simulink model "simL0_multiPath"  (R2024a)
settings: Solver=ode4  StartTime=0.0  StopTime=1500  FixedStep=0.01  MaxStep=0.01  MinStep=10^-3  RelTol=0.01
values from neighbouring files (symbols this model uses):
  MegAWESkite = yaml.ReadYaml('MegAWESkite.yaml',false,true)    [runMain.m]
undefined symbols (not defined in the file or in its folder): actuatorLimit, controllerGains_retraction, controllerGains_traction, DiscIntNeverNeededParam, ENVMT, pathparam, simInit, tetherParams, winchParameter
libraries: simulink x9, slpidlib x9, sharedtransform x3, aerolibutil x3, dspswit3 x2, dspinverses x2, shared6dof x1, simulink_extras x1, dspsigops x1, dspstat3 x1, vrlib x1
(part 3 of 5)

== system simL0_multiPath/Controls/RatesControl/rate controller/Pitch ==
  In1 : Inport
  In2 : Inport  Port=2
  Divide2 : Product  Inputs=*/
  Multiport Switch : MultiPortSwitch  SaturateOnIntegerOverflow=off  InputSameDT=off
  PID Controller : slpidlib/PID Controller  Controller=P  Form=Parallel  TimeDomain=Continuous-time  UseExternalTs=off  SampleTime=-1  IntegratorMethod=Forward Euler  FilterMethod=Forward Euler  ControllerParametersSource=internal  P=controllerGains_traction.ratePitch_P  I=1  UseKiTs=off  D=0  UseExternalDerivativeSource=off  N=100  UseFilter=on  TunerSelectOption=Transfer Function Based (PID Tuner App)  InitialConditionSource=internal  InitialConditionForIntegrator=0  InitialConditionForFilter=0  DifferentiatorICPrevScaledInput=0  ExternalReset=none  TrackingMode=off  Kt=1  LimitOutput=off  SatLimitsSource=internal  UpperSaturationLimit=inf  LowerSaturationLimit=-inf  LinearizeAsGain=on  AntiWindupMode=none  Kb=1  LimitIntegrator=off  UpperIntegratorSaturationLimit=inf  LowerIntegratorSaturationLimit=-inf  POutMin=[]  POutMax=[]  IOutMin=[]  IOutMax=[]  DOutMin=[]  DOutMax=[]  NOutMin=[]  NOutMax=[]  SumOutMin=[]  SumOutMax=[]  SaturationOutMin=[]  SaturationOutMax=[]  PParamMin=[]  PParamMax=[]  IParamMin=[]  IParamMax=[]  DParamMin=[]  DParamMax=[]  NParamMin=[]  NParamMax=[]  KbParamMin=[]  KbParamMax=[]  KtParamMin=[]  KtParamMax=[]  KbOutMin=[]  KbOutMax=[]  KtOutMin=[]  KtOutMax=[]  IntegratorOutMin=[]  IntegratorOutMax=[]  FilterOutMin=[]  FilterOutMax=[]  SumI1OutMin=[]  SumI1OutMax=[]  SumI2OutMin=[]  SumI2OutMax=[]  SumI3OutMin=[]  SumI3OutMax=[]  SumI4OutMin=[]  SumI4OutMax=[]  SumDOutMin=[]  SumDOutMax=[]  DifferentiatorOutMin=[]  DifferentiatorOutMax=[]  FilterDiffOutCoefMin=[]  FilterDiffOutCoefMax=[]  ReciprocalOutMin=[]  ReciprocalOutMax=[]  SumDenOutMin=[]  SumDenOutMax=[]  SumNumOutMin=[]  SumNumOutMax=[]  DivideOutMin=[]  DivideOutMax=[]  UdiffTsProdOutMin=[]  UdiffTsProdOutMax=[]  NTsProdOutMin=[]  NTsProdOutMax=[]  UintegralTsProdOutMin=[]  UintegralTsProdOutMax=[]  UngainTsProdOutMin=[]  UngainTsProdOutMax=[]  ClampingZeroOutDataTypeStr=Inherit: Inherit via back propagation  ClampingZeroOutMin=[]  ClampingZeroOutMax=[]  FilterDenConstantOutDataTypeStr=Inherit: Inherit via back propagation  FilterDenConstantOutMin=[]  FilterDenConstantOutMax=[]  PCopyOutDataTypeStr=Inherit: Inherit via back propagation  PCopyOutMin=[]  PCopyOutMax=[]  NCopyOutDataTypeStr=Inherit: Inherit via back propagation  NCopyOutMin=[]  NCopyOutMax=[]  IntegratorContinuousStateAttributes=''  IntegratorStateMustResolveToSignalObject=off  IntegratorRTWStateStorageClass=Auto  FilterContinuousStateAttributes=''  FilterStateMustResolveToSignalObject=off  FilterRTWStateStorageClass=Auto  ParallelPVariant=InternalParameters  IdealPVariant=Disabled  IVariant=Disabled  DVariant=Disabled  IntegratorVariant=Disabled  SatVariant=Disabled  AWVariant=Disabled  PCopyVariant=Disabled  TRVariant=Disabled  FdbkBlocksVariant=Forward  IdealPFdbkVariant=Disabled  SatFdbkVariant=Disabled  DerivativeFilterVariant=Disabled  NVariant=Disabled  NCopyVariant=Disabled_SignalSpec  FilterICVariant=Disabled  IntegratorICVariant=Disabled  ExternalResetVariant=Disabled  TRSumVariant=Passthrough  SumFdbkVariant=Disabled  SumVariant=Passthrough_P  TsampFilterVariant=InternalTs  TsampNgainVariant=Passthrough  TsampIntegralVariant=Disabled_SignalSpec  ExternalSaturationOutDataTypeStr=Inherit: Same as second input  DerivativeSourceVariant=Disabled
  PID Controller1 : slpidlib/PID Controller  Controller=P  Form=Parallel  TimeDomain=Continuous-time  UseExternalTs=off  SampleTime=-1  IntegratorMethod=Forward Euler  FilterMethod=Forward Euler  ControllerParametersSource=internal  P=controllerGains_retraction.ratePitch_P  I=1  UseKiTs=off  D=0  UseExternalDerivativeSource=off  N=100  UseFilter=on  TunerSelectOption=Transfer Function Based (PID Tuner App)  InitialConditionSource=internal  InitialConditionForIntegrator=0  InitialConditionForFilter=0  DifferentiatorICPrevScaledInput=0  ExternalReset=none  TrackingMode=off  Kt=1  LimitOutput=off  SatLimitsSource=internal  UpperSaturationLimit=inf  LowerSaturationLimit=-inf  LinearizeAsGain=on  AntiWindupMode=none  Kb=1  LimitIntegrator=off  UpperIntegratorSaturationLimit=inf  LowerIntegratorSaturationLimit=-inf  POutMin=[]  POutMax=[]  IOutMin=[]  IOutMax=[]  DOutMin=[]  DOutMax=[]  NOutMin=[]  NOutMax=[]  SumOutMin=[]  SumOutMax=[]  SaturationOutMin=[]  SaturationOutMax=[]  PParamMin=[]  PParamMax=[]  IParamMin=[]  IParamMax=[]  DParamMin=[]  DParamMax=[]  NParamMin=[]  NParamMax=[]  KbParamMin=[]  KbParamMax=[]  KtParamMin=[]  KtParamMax=[]  KbOutMin=[]  KbOutMax=[]  KtOutMin=[]  KtOutMax=[]  IntegratorOutMin=[]  IntegratorOutMax=[]  FilterOutMin=[]  FilterOutMax=[]  SumI1OutMin=[]  SumI1OutMax=[]  SumI2OutMin=[]  SumI2OutMax=[]  SumI3OutMin=[]  SumI3OutMax=[]  SumI4OutMin=[]  SumI4OutMax=[]  SumDOutMin=[]  SumDOutMax=[]  DifferentiatorOutMin=[]  DifferentiatorOutMax=[]  FilterDiffOutCoefMin=[]  FilterDiffOutCoefMax=[]  ReciprocalOutMin=[]  ReciprocalOutMax=[]  SumDenOutMin=[]  SumDenOutMax=[]  SumNumOutMin=[]  SumNumOutMax=[]  DivideOutMin=[]  DivideOutMax=[]  UdiffTsProdOutMin=[]  UdiffTsProdOutMax=[]  NTsProdOutMin=[]  NTsProdOutMax=[]  UintegralTsProdOutMin=[]  UintegralTsProdOutMax=[]  UngainTsProdOutMin=[]  UngainTsProdOutMax=[]  ClampingZeroOutDataTypeStr=Inherit: Inherit via back propagation  ClampingZeroOutMin=[]  ClampingZeroOutMax=[]  FilterDenConstantOutDataTypeStr=Inherit: Inherit via back propagation  FilterDenConstantOutMin=[]  FilterDenConstantOutMax=[]  PCopyOutDataTypeStr=Inherit: Inherit via back propagation  PCopyOutMin=[]  PCopyOutMax=[]  NCopyOutDataTypeStr=Inherit: Inherit via back propagation  NCopyOutMin=[]  NCopyOutMax=[]  IntegratorContinuousStateAttributes=''  IntegratorStateMustResolveToSignalObject=off  IntegratorRTWStateStorageClass=Auto  FilterContinuousStateAttributes=''  FilterStateMustResolveToSignalObject=off  FilterRTWStateStorageClass=Auto  ParallelPVariant=InternalParameters  IdealPVariant=Disabled  IVariant=Disabled  DVariant=Disabled  IntegratorVariant=Disabled  SatVariant=Disabled  AWVariant=Disabled  PCopyVariant=Disabled  TRVariant=Disabled  FdbkBlocksVariant=Forward  IdealPFdbkVariant=Disabled  SatFdbkVariant=Disabled  DerivativeFilterVariant=Disabled  NVariant=Disabled  NCopyVariant=Disabled_SignalSpec  FilterICVariant=Disabled  IntegratorICVariant=Disabled  ExternalResetVariant=Disabled  TRSumVariant=Passthrough  SumFdbkVariant=Disabled  SumVariant=Passthrough_P  TsampFilterVariant=InternalTs  TsampNgainVariant=Passthrough  TsampIntegralVariant=Disabled_SignalSpec  ExternalSaturationOutDataTypeStr=Inherit: Same as second input  DerivativeSourceVariant=Disabled
  Saturation : Saturate  UpperLimit=1  LowerLimit=-1  ZeroCross=off
  Scope : Scope
  Out1 : Outport  VectorParamsAs1DForOutWhenUnconnected=off
  wires:
  Saturation/1 -> Scope/1, Out1/1
  Divide2/1 -> Saturation/1
  In2/1 -> Divide2/2
  Multiport Switch/1 -> Divide2/1
  [F_state] -> Multiport Switch/1
  PID Controller/1 -> Multiport Switch/2, Multiport Switch/4
  PID Controller1/1 -> Multiport Switch/3
  In1/1 -> PID Controller1/1, PID Controller/1

== system simL0_multiPath/Controls/RatesControl/rate controller/Roll  ==
  In1 : Inport
  In2 : Inport  Port=2
  Divide2 : Product  Inputs=*/
  Multiport Switch : MultiPortSwitch  SaturateOnIntegerOverflow=off  InputSameDT=off
  PID Controller : slpidlib/PID Controller  Controller=P  Form=Parallel  TimeDomain=Continuous-time  UseExternalTs=off  SampleTime=-1  IntegratorMethod=Forward Euler  FilterMethod=Forward Euler  ControllerParametersSource=internal  P=controllerGains_traction.rateRoll_P  I=20  UseKiTs=off  D=1  UseExternalDerivativeSource=off  N=20  UseFilter=on  TunerSelectOption=Transfer Function Based (PID Tuner App)  InitialConditionSource=internal  InitialConditionForIntegrator=0  InitialConditionForFilter=0  DifferentiatorICPrevScaledInput=0  ExternalReset=none  TrackingMode=off  Kt=1  LimitOutput=off  SatLimitsSource=internal  UpperSaturationLimit=inf  LowerSaturationLimit=-inf  LinearizeAsGain=on  AntiWindupMode=none  Kb=1  LimitIntegrator=off  UpperIntegratorSaturationLimit=inf  LowerIntegratorSaturationLimit=-inf  POutMin=[]  POutMax=[]  IOutMin=[]  IOutMax=[]  DOutMin=[]  DOutMax=[]  NOutMin=[]  NOutMax=[]  SumOutMin=[]  SumOutMax=[]  SaturationOutMin=[]  SaturationOutMax=[]  PParamMin=[]  PParamMax=[]  IParamMin=[]  IParamMax=[]  DParamMin=[]  DParamMax=[]  NParamMin=[]  NParamMax=[]  KbParamMin=[]  KbParamMax=[]  KtParamMin=[]  KtParamMax=[]  KbOutMin=[]  KbOutMax=[]  KtOutMin=[]  KtOutMax=[]  IntegratorOutMin=[]  IntegratorOutMax=[]  FilterOutMin=[]  FilterOutMax=[]  SumI1OutMin=[]  SumI1OutMax=[]  SumI2OutMin=[]  SumI2OutMax=[]  SumI3OutMin=[]  SumI3OutMax=[]  SumI4OutMin=[]  SumI4OutMax=[]  SumDOutMin=[]  SumDOutMax=[]  DifferentiatorOutMin=[]  DifferentiatorOutMax=[]  FilterDiffOutCoefMin=[]  FilterDiffOutCoefMax=[]  ReciprocalOutMin=[]  ReciprocalOutMax=[]  SumDenOutMin=[]  SumDenOutMax=[]  SumNumOutMin=[]  SumNumOutMax=[]  DivideOutMin=[]  DivideOutMax=[]  UdiffTsProdOutMin=[]  UdiffTsProdOutMax=[]  NTsProdOutMin=[]  NTsProdOutMax=[]  UintegralTsProdOutMin=[]  UintegralTsProdOutMax=[]  UngainTsProdOutMin=[]  UngainTsProdOutMax=[]  ClampingZeroOutDataTypeStr=Inherit: Inherit via back propagation  ClampingZeroOutMin=[]  ClampingZeroOutMax=[]  FilterDenConstantOutDataTypeStr=Inherit: Inherit via back propagation  FilterDenConstantOutMin=[]  FilterDenConstantOutMax=[]  PCopyOutDataTypeStr=Inherit: Inherit via back propagation  PCopyOutMin=[]  PCopyOutMax=[]  NCopyOutDataTypeStr=Inherit: Inherit via back propagation  NCopyOutMin=[]  NCopyOutMax=[]  IntegratorContinuousStateAttributes=''  IntegratorStateMustResolveToSignalObject=off  IntegratorRTWStateStorageClass=Auto  FilterContinuousStateAttributes=''  FilterStateMustResolveToSignalObject=off  FilterRTWStateStorageClass=Auto  ParallelPVariant=InternalParameters  IdealPVariant=Disabled  IVariant=Disabled  DVariant=Disabled  IntegratorVariant=Disabled  SatVariant=Disabled  AWVariant=Disabled  PCopyVariant=Disabled  TRVariant=Disabled  FdbkBlocksVariant=Forward  IdealPFdbkVariant=Disabled  SatFdbkVariant=Disabled  DerivativeFilterVariant=Disabled  NVariant=Disabled  NCopyVariant=Disabled_SignalSpec  FilterICVariant=Disabled  IntegratorICVariant=Disabled  ExternalResetVariant=Disabled  TRSumVariant=Passthrough  SumFdbkVariant=Disabled  SumVariant=Passthrough_P  TsampFilterVariant=InternalTs  TsampNgainVariant=Passthrough  TsampIntegralVariant=Disabled_SignalSpec  ExternalSaturationOutDataTypeStr=Inherit: Same as second input  DerivativeSourceVariant=Disabled
  PID Controller1 : slpidlib/PID Controller  Controller=P  Form=Parallel  TimeDomain=Continuous-time  UseExternalTs=off  SampleTime=-1  IntegratorMethod=Forward Euler  FilterMethod=Forward Euler  ControllerParametersSource=internal  P=controllerGains_retraction.rateRoll_P  I=20  UseKiTs=off  D=1  UseExternalDerivativeSource=off  N=20  UseFilter=on  TunerSelectOption=Transfer Function Based (PID Tuner App)  InitialConditionSource=internal  InitialConditionForIntegrator=0  InitialConditionForFilter=0  DifferentiatorICPrevScaledInput=0  ExternalReset=none  TrackingMode=off  Kt=1  LimitOutput=off  SatLimitsSource=internal  UpperSaturationLimit=inf  LowerSaturationLimit=-inf  LinearizeAsGain=on  AntiWindupMode=none  Kb=1  LimitIntegrator=off  UpperIntegratorSaturationLimit=inf  LowerIntegratorSaturationLimit=-inf  POutMin=[]  POutMax=[]  IOutMin=[]  IOutMax=[]  DOutMin=[]  DOutMax=[]  NOutMin=[]  NOutMax=[]  SumOutMin=[]  SumOutMax=[]  SaturationOutMin=[]  SaturationOutMax=[]  PParamMin=[]  PParamMax=[]  IParamMin=[]  IParamMax=[]  DParamMin=[]  DParamMax=[]  NParamMin=[]  NParamMax=[]  KbParamMin=[]  KbParamMax=[]  KtParamMin=[]  KtParamMax=[]  KbOutMin=[]  KbOutMax=[]  KtOutMin=[]  KtOutMax=[]  IntegratorOutMin=[]  IntegratorOutMax=[]  FilterOutMin=[]  FilterOutMax=[]  SumI1OutMin=[]  SumI1OutMax=[]  SumI2OutMin=[]  SumI2OutMax=[]  SumI3OutMin=[]  SumI3OutMax=[]  SumI4OutMin=[]  SumI4OutMax=[]  SumDOutMin=[]  SumDOutMax=[]  DifferentiatorOutMin=[]  DifferentiatorOutMax=[]  FilterDiffOutCoefMin=[]  FilterDiffOutCoefMax=[]  ReciprocalOutMin=[]  ReciprocalOutMax=[]  SumDenOutMin=[]  SumDenOutMax=[]  SumNumOutMin=[]  SumNumOutMax=[]  DivideOutMin=[]  DivideOutMax=[]  UdiffTsProdOutMin=[]  UdiffTsProdOutMax=[]  NTsProdOutMin=[]  NTsProdOutMax=[]  UintegralTsProdOutMin=[]  UintegralTsProdOutMax=[]  UngainTsProdOutMin=[]  UngainTsProdOutMax=[]  ClampingZeroOutDataTypeStr=Inherit: Inherit via back propagation  ClampingZeroOutMin=[]  ClampingZeroOutMax=[]  FilterDenConstantOutDataTypeStr=Inherit: Inherit via back propagation  FilterDenConstantOutMin=[]  FilterDenConstantOutMax=[]  PCopyOutDataTypeStr=Inherit: Inherit via back propagation  PCopyOutMin=[]  PCopyOutMax=[]  NCopyOutDataTypeStr=Inherit: Inherit via back propagation  NCopyOutMin=[]  NCopyOutMax=[]  IntegratorContinuousStateAttributes=''  IntegratorStateMustResolveToSignalObject=off  IntegratorRTWStateStorageClass=Auto  FilterContinuousStateAttributes=''  FilterStateMustResolveToSignalObject=off  FilterRTWStateStorageClass=Auto  ParallelPVariant=InternalParameters  IdealPVariant=Disabled  IVariant=Disabled  DVariant=Disabled  IntegratorVariant=Disabled  SatVariant=Disabled  AWVariant=Disabled  PCopyVariant=Disabled  TRVariant=Disabled  FdbkBlocksVariant=Forward  IdealPFdbkVariant=Disabled  SatFdbkVariant=Disabled  DerivativeFilterVariant=Disabled  NVariant=Disabled  NCopyVariant=Disabled_SignalSpec  FilterICVariant=Disabled  IntegratorICVariant=Disabled  ExternalResetVariant=Disabled  TRSumVariant=Passthrough  SumFdbkVariant=Disabled  SumVariant=Passthrough_P  TsampFilterVariant=InternalTs  TsampNgainVariant=Passthrough  TsampIntegralVariant=Disabled_SignalSpec  ExternalSaturationOutDataTypeStr=Inherit: Same as second input  DerivativeSourceVariant=Disabled
  Saturation : Saturate  UpperLimit=1  LowerLimit=-1  ZeroCross=off
  Out1 : Outport  VectorParamsAs1DForOutWhenUnconnected=off
  wires:
  Saturation/1 -> Out1/1
  Divide2/1 -> Saturation/1
  In2/1 -> Divide2/2
  In1/1 -> PID Controller/1, PID Controller1/1
  [F_state] -> Multiport Switch/1
  PID Controller1/1 -> Multiport Switch/3
  Multiport Switch/1 -> Divide2/1
  PID Controller/1 -> Multiport Switch/2, Multiport Switch/4

== system simL0_multiPath/Controls/RatesControl/rate controller/Yaw ==
  In1 : Inport
  In2 : Inport  Port=2
  Divide2 : Product  Inputs=*/
  Multiport Switch : MultiPortSwitch  SaturateOnIntegerOverflow=off  InputSameDT=off
  PID Controller : simulink/Continuous/PID Controller  Controller=P  Form=Parallel  TimeDomain=Continuous-time  SampleTime=-1  IntegratorMethod=Forward Euler  FilterMethod=Forward Euler  ControllerParametersSource=internal  P=controllerGains_traction.rateYaw_P  I=20  D=1  UseFilter=on  N=20  TunerSelectOption=Transfer Function Based (PID Tuner App)  InitialConditionSource=internal  InitialConditionForIntegrator=0  InitialConditionForFilter=0  DifferentiatorICPrevScaledInput=0  ExternalReset=none  TrackingMode=off  Kt=1  LimitOutput=off  UpperSaturationLimit=inf  LowerSaturationLimit=-inf  LinearizeAsGain=on  AntiWindupMode=none  Kb=1  POutMin=[]  POutMax=[]  IOutMin=[]  IOutMax=[]  DOutMin=[]  DOutMax=[]  NOutMin=[]  NOutMax=[]  SumOutMin=[]  SumOutMax=[]  SaturationOutMin=[]  SaturationOutMax=[]  PParamMin=[]  PParamMax=[]  IParamMin=[]  IParamMax=[]  DParamMin=[]  DParamMax=[]  NParamMin=[]  NParamMax=[]  KbParamMin=[]  KbParamMax=[]  KtParamMin=[]  KtParamMax=[]  KbOutMin=[]  KbOutMax=[]  KtOutMin=[]  KtOutMax=[]  IntegratorOutMin=[]  IntegratorOutMax=[]  FilterOutMin=[]  FilterOutMax=[]  SumI1OutMin=[]  SumI1OutMax=[]  SumI2OutMin=[]  SumI2OutMax=[]  SumI3OutMin=[]  SumI3OutMax=[]  SumI4OutMin=[]  SumI4OutMax=[]  SumDOutMin=[]  SumDOutMax=[]  DifferentiatorOutMin=[]  DifferentiatorOutMax=[]  FilterDiffOutCoefMin=[]  FilterDiffOutCoefMax=[]  ReciprocalOutMin=[]  ReciprocalOutMax=[]  SumDenOutMin=[]  SumDenOutMax=[]  SumNumOutMin=[]  SumNumOutMax=[]  DivideOutMin=[]  DivideOutMax=[]  IntegratorContinuousStateAttributes=''  IntegratorStateMustResolveToSignalObject=off  IntegratorRTWStateStorageClass=Auto  FilterContinuousStateAttributes=''  FilterStateMustResolveToSignalObject=off  FilterRTWStateStorageClass=Auto  ParallelPVariant=InternalParameters  IdealPVariant=Disabled  IVariant=Disabled  DVariant=Disabled  IntegratorVariant=Disabled  SatVariant=Disabled  AWVariant=Disabled  PCopyVariant=Disabled  TRVariant=Disabled  FdbkBlocksVariant=Forward  IdealPFdbkVariant=Disabled  SatFdbkVariant=Disabled  DerivativeFilterVariant=Disabled  NVariant=Disabled  NCopyVariant=Disabled_SignalSpec  FilterICVariant=Disabled  IntegratorICVariant=Disabled  ExternalResetVariant=Disabled  TRSumVariant=Passthrough  SumFdbkVariant=Disabled  SumVariant=Passthrough_P
  PID Controller1 : simulink/Continuous/PID Controller  Controller=P  Form=Parallel  TimeDomain=Continuous-time  SampleTime=-1  IntegratorMethod=Forward Euler  FilterMethod=Forward Euler  ControllerParametersSource=internal  P=controllerGains_retraction.rateYaw_P  I=20  D=1  UseFilter=on  N=20  TunerSelectOption=Transfer Function Based (PID Tuner App)  InitialConditionSource=internal  InitialConditionForIntegrator=0  InitialConditionForFilter=0  DifferentiatorICPrevScaledInput=0  ExternalReset=none  TrackingMode=off  Kt=1  LimitOutput=off  UpperSaturationLimit=inf  LowerSaturationLimit=-inf  LinearizeAsGain=on  AntiWindupMode=none  Kb=1  POutMin=[]  POutMax=[]  IOutMin=[]  IOutMax=[]  DOutMin=[]  DOutMax=[]  NOutMin=[]  NOutMax=[]  SumOutMin=[]  SumOutMax=[]  SaturationOutMin=[]  SaturationOutMax=[]  PParamMin=[]  PParamMax=[]  IParamMin=[]  IParamMax=[]  DParamMin=[]  DParamMax=[]  NParamMin=[]  NParamMax=[]  KbParamMin=[]  KbParamMax=[]  KtParamMin=[]  KtParamMax=[]  KbOutMin=[]  KbOutMax=[]  KtOutMin=[]  KtOutMax=[]  IntegratorOutMin=[]  IntegratorOutMax=[]  FilterOutMin=[]  FilterOutMax=[]  SumI1OutMin=[]  SumI1OutMax=[]  SumI2OutMin=[]  SumI2OutMax=[]  SumI3OutMin=[]  SumI3OutMax=[]  SumI4OutMin=[]  SumI4OutMax=[]  SumDOutMin=[]  SumDOutMax=[]  DifferentiatorOutMin=[]  DifferentiatorOutMax=[]  FilterDiffOutCoefMin=[]  FilterDiffOutCoefMax=[]  ReciprocalOutMin=[]  ReciprocalOutMax=[]  SumDenOutMin=[]  SumDenOutMax=[]  SumNumOutMin=[]  SumNumOutMax=[]  DivideOutMin=[]  DivideOutMax=[]  IntegratorContinuousStateAttributes=''  IntegratorStateMustResolveToSignalObject=off  IntegratorRTWStateStorageClass=Auto  FilterContinuousStateAttributes=''  FilterStateMustResolveToSignalObject=off  FilterRTWStateStorageClass=Auto  ParallelPVariant=InternalParameters  IdealPVariant=Disabled  IVariant=Disabled  DVariant=Disabled  IntegratorVariant=Disabled  SatVariant=Disabled  AWVariant=Disabled  PCopyVariant=Disabled  TRVariant=Disabled  FdbkBlocksVariant=Forward  IdealPFdbkVariant=Disabled  SatFdbkVariant=Disabled  DerivativeFilterVariant=Disabled  NVariant=Disabled  NCopyVariant=Disabled_SignalSpec  FilterICVariant=Disabled  IntegratorICVariant=Disabled  ExternalResetVariant=Disabled  TRSumVariant=Passthrough  SumFdbkVariant=Disabled  SumVariant=Passthrough_P
  Saturation : Saturate  UpperLimit=1  LowerLimit=-1  ZeroCross=off
  Out1 : Outport  VectorParamsAs1DForOutWhenUnconnected=off
  wires:
  In2/1 -> Divide2/2
  Divide2/1 -> Saturation/1
  Saturation/1 -> Out1/1
  Multiport Switch/1 -> Divide2/1
  [F_state] -> Multiport Switch/1
  PID Controller/1 -> Multiport Switch/2, Multiport Switch/4
  PID Controller1/1 -> Multiport Switch/3
  In1/1 -> PID Controller1/1, PID Controller/1

== stateflow chart simL0_multiPath/Computer 1/Chart ==
  state Traction_phase
    flightState=1;
  note: up loop
  note: down loop
  state Transition_phase_retract_to_tract
    flightState=3;
  note: cirlce
  state Retraction_phase
    flightState=2;
  state Transition_phase_tract_to_retract
    flightState=1;
  note: up loop
  note: down loop
  note: cirlce
  (junction 46) -> Traction_phase : [numPatterns>=1]
  Traction_phase -> (junction 46) [order 2] : [numPatterns==0]
  (default) -> Traction_phase
  Transition_phase_retract_to_tract -> Traction_phase [order 2] : [~pathparam.isCircle && pathparam.direction<0 && (s_path >4*pi/3 && s_path< 2*pi )]
  Transition_phase_retract_to_tract -> Traction_phase [order 1] : [~pathparam.isCircle && pathparam.direction>0 && (s_path >pi/2 && s_path< 3*pi/2 )]
  Transition_phase_retract_to_tract -> Traction_phase [order 3] : [pathparam.isCircle && (s_path >=pi/2 && s_path< 3*pi/2 )]
  Retraction_phase -> Transition_phase_retract_to_tract : [tetherLength<tetherParams.minLength*tetherParams.maxLength || kitePos(1)<retractTarget(1)]
  Traction_phase -> Transition_phase_tract_to_retract [order 1] : [tetherLength>tetherParams.maxLength]
  Transition_phase_tract_to_retract -> Retraction_phase [order 2] : [~pathparam.isCircle && pathparam.direction<0 && (s_path >pi/2 && s_path< 2*pi/3 )]
  Transition_phase_tract_to_retract -> Retraction_phase [order 1] : [~pathparam.isCircle && pathparam.direction>0 && (s_path >= 0 && s_path < pi/10)]
  Transition_phase_tract_to_retract -> Retraction_phase [order 3] : [pathparam.isCircle && (s_path >= 4*pi/3 && s_path < 5*pi/3)]
  data: numPatterns input; flightState output =1; tetherLength input; kitePos input; retractTarget constant double size=[3,1] =pathparam.retractionTarget; s_path input; pathparam parameter; tetherParams parameter

== matlab function simL0_multiPath/ParticleTetherModel/Tether_Dynamics1 ==
  data: kitePos input; tetherPos output size=[3,tetherParams.numParticles]; kiteVel input; windVel input; tetherLength input; x input; Ft_Ground output; Ft_Kite output; Fobj output; exitFlag output; x output; ENVMT parameter; tetherParams parameter
% Copyright 2021 Delft University of Technology
%
% Licensed under the Apache License, Version 2.0 (the "License");
% you may not use this file except in compliance with the License.
% You may obtain a copy of the License at
%
%      http://www.apache.org/licenses/LICENSE-2.0
%
% Unless required by applicable law or agreed to in writing, software
% distributed under the License is distributed on an "AS IS" BASIS,
% WITHOUT WARRANTIES OR CONDITIONS OF ANY KIND, either express or implied.
% See the License for the specific language governing permissions and
% limitations under the License.

function [tetherPos, Ft_Ground, Ft_Kite, Fobj, exitFlag, x]= ...
    Tether_QuasiStatic(kitePos, kiteVel, windVel, tetherLength, x,ENVMT,tetherParams)
%#codegen

%Tether_QuasiStatic Trust-region dogleg nonlinear systems of equation
%   solver to determine the tether shape and forces.
%
%   Tether_QuasiStatic is based on the matlab implementation that 
%   solves a system of nonlinear equations using a dogleg
%   trust region approach.  The algorithm implemented is similar in nature
%   to the FORTRAN program HYBRD1 of J.J. More', B.S. Garbow and K.E. 
%   Hillstrom, User Guide for MINPACK 1, Argonne National Laboratory, 
%   Rept. ANL-80-74, 1980, which itself was based on the program CALFUN 
%   of M.J.D. Powell, A Fortran subroutine for solving systems of
%   nonlinear algebraic equations, Chap. 7 in P. Rabinowitz, ed.,
%   Numerical Methods for Nonlinear Algebraic Equations, Gordon and
%   Breach, New York, 1970.
%
%   Addapted by Ir. D. Eijkelhof (TU Delft) from 1990-2019 Matlab version 
%   The MathWorks, Inc.
% NOTE: From Matlab 2020b Matlab's Levenberg–Marquardt algorithm in the
% command "solve" can be directly used in codegen and might be
% faster. Due to availability of only matlab R2019B and lower, an own
% implementation had to be used in order the execute codegen.
%
% Syntax:  [tetherPos, Ft_Ground, Ft_Kite, Fvec, x]= ...
%     Tether_QuasiStatic(kitePos, kiteVel, windVel, tetherLength, x, ENVMT, T)
%
% NOTE: 'x' passed in and returned in column vector form.
%
% Throughout this routine 'x', 'F', 'xvec', 'xTrial', 'Fvec' and 'FTrial' are vectors.
%
% Inputs:
%    tetherPos  - Position vectors of tether particles
%    Ft_Ground  - Tether force magnitude at the ground station
%    Ft_Kite    - Tether force vector at the kite
%    Fvec       - Error between tether end and kite position (3D)
%    x          - Tether ground segment orientation and magnitude
%
% Outputs:
%    kitePos        - Kite position vector in wind reference frame
%    kiteVel        - Kite velocity vector in wind reference frame
%    windVel        - Wind velocity vector in wind reference frame
%    ENVMT          - Environmental parameters
%    tetherLength   - Reeled-out tether length determined by the winch
%    x              - Initial tether ground segment orientation and magnitude
%    T              - Tether dimensions and material properties
%
% Other m-files required: none
%
% Subfunctions: Objfunc    : Calculate difference between tether end and
%                            kite given tether ground segment orientation
%                            and magnitude.
%               testStop   : Test convergence criteria's
%               dogleg_tem : approximately solves trust region subproblem
%                            via a dogleg approach. 
%               lm_FD_J    : Determines the jacobian matrix by forward
%                            differencing
%
% MAT-files required: none
%
% Author: Dylan Eijkelhof, M.Sc.
% Delft University of Technology
% email address: d.eijkelhof@tudelft.nl  
% December 2019; Last revision: 16-March-2021

%------------- BEGIN CODE --------------

    % fun = @(x) Objfunc(x,kitePos,kiteVel,windVel,tetherLength,ENVMT,tetherParams);
    fun = @(x) norm(Objfunc(x,kitePos,kiteVel,windVel,tetherLength,ENVMT,tetherParams))^2;

    options = optimoptions('fsolve','Algorithm','levenberg-marquardt',...
        'Display','none',...
        'MaxIterations',2000,...
        'MaxFunctionEvaluations',1000, ...
        'StepTolerance',1e-12,...
        'FiniteDifferenceStepSize',1e-6,...
        'FiniteDifferenceType','central');
    [x,~,exitFlag,~,~] = fsolve(fun,x,options);
    % fun = @(x) norm(Objfunc(x,kitePos,kiteVel,windVel,tetherLength,ENVMT,tetherParams))^2;
    % 
    % options = optimoptions('fmincon','Algorithm','sqp','Display','final',...
    % 'MaxIterations',2000,...
    % 'MaxFunctionEvaluations',1000, ...
    % 'OptimalityTolerance',1e-12,...
    % 'StepTolerance',1e-12,...
    % 'ConstraintTolerance',1e-12,...
    % 'FiniteDifferenceStepSize',1e-6,...
    % 'FiniteDifferenceType','central');
    % 
    % 
    % lb = [0, -pi/2, 0]; % Lower bounds
    % ub = [pi/2, pi/2, Inf]; % Upper bounds
    % 
    % [x,~,exitFlag] = fmincon(fun,x,[],[],[],[],lb,ub,[],options);

    [Fobj,T0,pj,~] = Objfunc(x,kitePos, kiteVel, windVel,...
                              tetherLength, ENVMT, tetherParams);

    % Optimization is finished.  
    Ft_Ground   = x(3);
    Ft_Kite     = T0;
    tetherPos   = pj;
end


function [Fobj,T0,pj,p0] = Objfunc(stateVec,kitePos, kiteVel, windVel,...
                              tetherLength, ENVMT, T)
    Ns = size(windVel,2);       % number of masses
    Ls = tetherLength/(Ns+1);   % segment length
    mj = T.rho_t * Ls;          % segment mass

    p = kitePos;                % input aircraft position
    v = kiteVel;                % input aircraft velocity

    theta = stateVec(1);
    phi = stateVec(2);
    Tn = stateVec(3);

    omega_t = cross(p./(norm(p)^2),v);

    E = T.modulusE;
    A = T.A;

    FT = zeros(3,Ns); % Tension forces
    Fd = zeros(3,Ns); % Drag forces
    pj = zeros(3,Ns); % Mass positions
    vj = zeros(3,Ns); % Mass velocities
    aj = zeros(3,Ns); % Mass accellerations

    % First element from ground station (Ns)
    % FT(:,Ns) = Tn.*[sin(theta)* cos(phi); sin(phi); cos(theta)*cos(phi)];
    % pj(:,Ns) = Ls.*[sin(theta)* cos(phi); sin(phi); cos(theta)*cos(phi)];
    rotVec=[cos(theta)* cos(phi); sin(theta)* cos(phi); sin(phi)];
    FT(:,Ns) = Tn.*rotVec;
    pj(:,Ns) = Ls.*rotVec;

    vj(:,Ns) = dot(v,p./norm(p)) .* (p./norm(p)) + cross(omega_t,pj(:,Ns));
    aj(:,Ns) = cross(omega_t,cross(omega_t,pj(:,Ns)));
    
    % Drag calculation first element
    v_a_p = vj(:,Ns) - windVel(:,Ns);
    if all(abs(v_a_p)<1e-3)
        Fd(:,Ns) = [0;0;0];
    else
        v_a_p_t = dot((pj(:,Ns))/norm(pj(:,Ns)),v_a_p)*...
            ((pj(:,Ns))/norm(pj(:,Ns)));
        v_a_p_n = v_a_p - v_a_p_t;
        Fd(:,Ns) = -0.5 * ENVMT.rhos * Ls * T.d_tether * T.CD * ...
            norm(v_a_p_n) * v_a_p_n; % particle drag
    end
    
    % All other segments and masses except for segment connected to the kite
    for i = Ns:-1:2
        if i == Ns
            FT(:,i-1) = (mj+0.5*mj).*aj(:,i) + FT(:,i) - Fd(:,i) + ...
                [0;0;(mj+0.5*mj)*ENVMT.g];
        else
            FT(:,i-1) = mj.*aj(:,i) + FT(:,i) - Fd(:,i) + [0;0;mj*ENVMT.g];
        end

        l_i_1 = (norm(FT(:,i-1))/(E*A) + 1)*Ls;
        
        pj(:,i-1) = pj(:,i) + l_i_1.*(FT(:,i-1)/norm(FT(:,i-1)));       
        vj(:,i-1) = dot(v,p./norm(p)) .* (p./norm(p)) + cross(omega_t,pj(:,i-1));
        aj(:,i-1) = cross(omega_t,cross(omega_t,pj(:,i-1)));
        
        % Drag calculation
        v_a_p = vj(:,i) - windVel(:,i);
        if all(abs(v_a_p)<1e-3)
            Fd(:,i-1) = [0;0;0];
        else
            v_a_p_t = dot((pj(:,i-1)-pj(:,i))/norm(pj(:,i-1)-pj(:,i)),v_a_p) * ...
                ((pj(:,i-1)-pj(:,i))/norm(pj(:,i-1)-pj(:,i)));
            v_a_p_n = v_a_p - v_a_p_t;
            Fd(:,i-1) = -0.5 * ENVMT.rhos * Ls * T.d_tether * T.CD * ...
                norm(v_a_p_n) * v_a_p_n; % particle drag
        end
    end
    
    T0 = (mj+0.5*mj).*aj(:,1) + FT(:,1) - Fd(:,1) + [0;0;(mj+0.5*mj)*ENVMT.g];
    l_i_1 = (norm(T0)/(E*A) + 1)*Ls;
    p0 = pj(:,1) + l_i_1.*(T0/norm(T0));
    
    Fobj = p-p0;
end

== matlab function simL0_multiPath/Output/MATLAB Function1 ==
  data: u input; y output
function y = fcn(u)

y = atan2(u(3),u(1));

== matlab function simL0_multiPath/Controls/ FlightControl/traction/Convert YPR-tantoe1 ==
  data: input input; roll output; pitch output; yaw output
%Function that convert Euler angles from actual tangential ref to earth

function [roll,pitch, yaw] = YPR_convert_tantoe(input)

%Aircraft position coordinates in earth ref system
x_a = input(1);
y_a = input(2);
z_a = input(3); 

[azi, el, r] = cart2sph(x_a,y_a,z_a); %Convert into spherical coordiantes
el = -el;            %Adjust to the definition positive elev angle pointing upwards
azi = -azi +pi/2;

%Aircraft euler rotation angles wrt to earth ref system
a_roll    = input(4);
a_pitch   = input(5);
a_yaw     = input(6);

%R_e = fromEuler(yaw, pitch, roll) -> define the rotation Rz*Ry*Rx
a_x = a_roll;
a_y = a_pitch;
a_z = a_yaw;

R = [cos(a_y)*cos(a_z), sin(a_x)*sin(a_y)*cos(a_z)-cos(a_x)*sin(a_z), cos(a_x)*sin(a_y)*cos(a_z)+sin(a_x)*sin(a_z);
     cos(a_y)*sin(a_z), sin(a_x)*sin(a_y)*sin(a_z)+cos(a_x)*cos(a_z), cos(a_x)*sin(a_y)*sin(a_z)-sin(a_x)*cos(a_z);
     -sin(a_y), sin(a_x)*cos(a_y), cos(a_x)*cos(a_y)];
 
%Building transformation matrix form eart to tan ref frame 
a_x = -el;
a_y = 0;
a_z = -azi;

R_1 = [cos(a_y)*cos(a_z), sin(a_x)*sin(a_y)*cos(a_z)-cos(a_x)*sin(a_z), cos(a_x)*sin(a_y)*cos(a_z)+sin(a_x)*sin(a_z);
     cos(a_y)*sin(a_z), sin(a_x)*sin(a_y)*sin(a_z)+cos(a_x)*cos(a_z), cos(a_x)*sin(a_y)*sin(a_z)-sin(a_x)*cos(a_z);
     -sin(a_y), sin(a_x)*cos(a_y), cos(a_x)*cos(a_y)];
 
a_x = 0;
a_y = pi/2;
a_z = -pi/2;  %Adjusted to obtain NED direction
 
R_2 = [cos(a_y)*cos(a_z), sin(a_x)*sin(a_y)*cos(a_z)-cos(a_x)*sin(a_z), cos(a_x)*sin(a_y)*cos(a_z)+sin(a_x)*sin(a_z);
     cos(a_y)*sin(a_z), sin(a_x)*sin(a_y)*sin(a_z)+cos(a_x)*cos(a_z), cos(a_x)*sin(a_y)*sin(a_z)-sin(a_x)*cos(a_z);
     -sin(a_y), sin(a_x)*cos(a_y), cos(a_x)*cos(a_y)];
 
R_etotan = R_1*R_2; %Earth to tan
R_tantoe = inv(R_etotan);

R_relativ=((R_tantoe)'*R);

%Extract euler Angles 
eul_l_p = zeros(1,3);
eul_l_p(2)=asin(-R_relativ(3,1));
if abs(eul_l_p(2)-pi/2)<1e-3
    eul_l_p(1)=0;
    eul_l_p(3)=atan2(R_relativ(2,3) - R_relativ(1,2),R_relativ(1,3)+R_relativ(2,2)+eul_l_p(1));
elseif abs(eul_l_p(2)+pi/2)<1e-3
    eul_l_p(1)=0;
    eul_l_p(3)=atan2(R_relativ(2,3) - R_relativ(1,2),R_relativ(1,3)+R_relativ(2,2)+eul_l_p(1));
else
    eul_l_p(1)=atan2(R_relativ(3,2),R_relativ(3,3));
    eul_l_p(3)=atan2(R_relativ(2,1),R_relativ(1,1));
end

roll = eul_l_p(1);                            
pitch = eul_l_p(2);  
yaw = eul_l_p(3);

end

== matlab function simL0_multiPath/Controls/ FlightControl/Convert YPR-tantoe ==
  data: input input; roll output; pitch output; yaw output
%Function that convert Euler angles from actual tangential ref to earth

function [roll,pitch, yaw] = YPR_convert_tantoe(input)

%Aircraft position coordinates in earth ref system
x_a = input(1);
y_a = input(2);
z_a = input(3); 

[azi, el, r] = cart2sph(x_a,y_a,z_a); %Convert into spherical coordiantes
el = -el;            %Adjust to the definition positive elev angle pointing upwards
azi = -azi +pi/2;

%Aircraft euler rotation angles wrt to earth ref system
a_roll    = input(4);
a_pitch   = input(5);
a_yaw     = input(6);

%R_e = fromEuler(yaw, pitch, roll) -> define the rotation Rz*Ry*Rx
a_x = a_roll;
a_y = a_pitch;
a_z = a_yaw;

R = [cos(a_y)*cos(a_z), sin(a_x)*sin(a_y)*cos(a_z)-cos(a_x)*sin(a_z), cos(a_x)*sin(a_y)*cos(a_z)+sin(a_x)*sin(a_z);
     cos(a_y)*sin(a_z), sin(a_x)*sin(a_y)*sin(a_z)+cos(a_x)*cos(a_z), cos(a_x)*sin(a_y)*sin(a_z)-sin(a_x)*cos(a_z);
     -sin(a_y), sin(a_x)*cos(a_y), cos(a_x)*cos(a_y)];
 
%Building transformation matrix form eart to tan ref frame 
a_x = -el;
a_y = 0;
a_z = -azi;

R_1 = [cos(a_y)*cos(a_z), sin(a_x)*sin(a_y)*cos(a_z)-cos(a_x)*sin(a_z), cos(a_x)*sin(a_y)*cos(a_z)+sin(a_x)*sin(a_z);
     cos(a_y)*sin(a_z), sin(a_x)*sin(a_y)*sin(a_z)+cos(a_x)*cos(a_z), cos(a_x)*sin(a_y)*sin(a_z)-sin(a_x)*cos(a_z);
     -sin(a_y), sin(a_x)*cos(a_y), cos(a_x)*cos(a_y)];
 
a_x = 0;
a_y = pi/2;
a_z = -pi/2;  %Adjusted to obtain NED direction
 
R_2 = [cos(a_y)*cos(a_z), sin(a_x)*sin(a_y)*cos(a_z)-cos(a_x)*sin(a_z), cos(a_x)*sin(a_y)*cos(a_z)+sin(a_x)*sin(a_z);
     cos(a_y)*sin(a_z), sin(a_x)*sin(a_y)*sin(a_z)+cos(a_x)*cos(a_z), cos(a_x)*sin(a_y)*sin(a_z)-sin(a_x)*cos(a_z);
     -sin(a_y), sin(a_x)*cos(a_y), cos(a_x)*cos(a_y)];
 
R_etotan = R_1*R_2; %Earth to tan
R_tantoe = inv(R_etotan);

R_relativ=((R_tantoe)'*R);

%Extract euler Angles 
eul_l_p = zeros(1,3);
eul_l_p(2)=asin(-R_relativ(3,1));
if abs(eul_l_p(2)-pi/2)<1e-3
    eul_l_p(1)=0;
    eul_l_p(3)=atan2(R_relativ(2,3) - R_relativ(1,2),R_relativ(1,3)+R_relativ(2,2)+eul_l_p(1));
elseif abs(eul_l_p(2)+pi/2)<1e-3
    eul_l_p(1)=0;
    eul_l_p(3)=atan2(R_relativ(2,3) - R_relativ(1,2),R_relativ(1,3)+R_relativ(2,2)+eul_l_p(1));
else
    eul_l_p(1)=atan2(R_relativ(3,2),R_relativ(3,3));
    eul_l_p(3)=atan2(R_relativ(2,1),R_relativ(1,1));
end

roll = eul_l_p(1);                            
pitch = eul_l_p(2);  
yaw = eul_l_p(3);

end

== matlab function simL0_multiPath/Controls/ FlightControl/Path_8_sim_v4 ==
  data: target_p output; a_posW input; closest_p output; s_cnew output; s_targ output; d_l1 output; dist_p output; np_ahead input; pathparam parameter
% PATH-FOLLOWING-BLOCK_ FIGURE_OF_EIGHT 

%Description: This block implements the figure of eight path following
%             generating the desidered path in sphere as set of points 
%            
%             Determines the target point coordinates and closest point 
%             to the current aircraft position and both relative s value
%             on the path

function [target_p,closest_p,s_cnew,s_targ,d_l1,dist_p] = path(a_posW,np_ahead, pathparam)

persistent c_i_prev;
if isempty(c_i_prev)    %Index of the s vector to previous closest point
    c_i_prev = 25;      
end  

phi_el = pathparam.elevAng;
theta  = pathparam.polarAng;

abooth = pathparam.aBooth;
bbooth = pathparam.bBooth;
htau = pathparam.hTau;

k = pathparam.direction;
% negative: up loop or anti-clockwise 
% positive down loop or clockwise


R = sqrt(a_posW(1).^2 + a_posW(2).^2 + a_posW(3).^2);

xc =  R * cos(phi_el)*cos(theta);      
yc =  R * cos(phi_el)*sin(theta);       %Center of the circle path
zc =  R * sin(phi_el);

pc = [xc,yc,zc];

% Define the normal vector to the plane aligned 
% with the vector btw center (ground station) and center of circle path
vc = [xc,yc,zc];
vc_n = vc/norm(vc); %down

% Choose two non-parallel vectors in the plane 
u = [-cos(phi_el)*cos(theta),cos(phi_el)*sin(theta),sin(phi_el)]; 

% Take the cross product of the two vectors to get a vector orthogonal to the plane 
v = cross(u, vc_n);

% NED basis for the plane
e1 = v / norm(u);   %E
e2 = u / norm(v);   %N
e3 = -vc_n;         %D


% Define the range of s values
s = linspace(0,sign(k)*2*pi,50);           % (-) 2*pi to follow flight path in right direction


% Function to generate Figure-of-eight path
function [xP,yP,zP] = gen_path8(s,e1,e2,pc,R)
    
    x_s = 1/htau * bbooth * sin(s) ./ (1 + (abooth/bbooth)^2 * cos(s).^2);
    y_s = 1/htau* abooth * sin(s) .* cos(s) ./ (1 + (abooth/bbooth)^2 * cos(s).^2);

    x = pc(1) + x_s * e1(1) + y_s * e2(1);
    y = pc(2) + x_s * e1(2) + y_s * e2(2);  % Path moved tangent to flight sphere
    z = pc(3) + x_s * e1(3) + y_s * e2(3);   

    xP = real(R * x./ sqrt(x.^2 + y.^2 + z.^2));
    yP = real(R * y./ sqrt(x.^2 + y.^2 + z.^2));  %Projection path on the sphere
    zP = real(R * z./ sqrt(x.^2 + y.^2 + z.^2));

end

[xP,yP,zP] = gen_path8(s,e1,e2,pc,R);    %Generate the path [matrix coordinates]
path = [xP;yP;zP];

%Calculates the distances from airc pos to every point on the path
d_to_p = sqrt((path(1,:) - a_posW(1)).^2 + (path(2,:) - a_posW(2)).^2 + (path(3,:) - a_posW(3)).^2);


%Generate a circular vector of distances shifted in such a way that the
%first element 
d_to_p_shift = circshift(d_to_p,-c_i_prev+8);  
d_to_p_shift = d_to_p_shift(1:25);            %Consider only 25 elems (half of the path)

[dist_p,i_d] = min(d_to_p_shift);      %Find index with minimum lenght

i_cnew = i_d + c_i_prev -8;       %Find the right index wrt s

if i_cnew <=0
    i_cnew = i_cnew + length(s);
end

if i_cnew >length(s)
   i_cnew = i_cnew - length(s);
end

c_i_prev = i_cnew;      %Update previuos closest index for next iteration
s_cnew = s(i_cnew);     %Calculates the corresponding s value of the index


[xC,yC,zC] = gen_path8(s_cnew,e1,e2,pc,R);        %Generate the closest point
closest_p = [xC,yC,zC];

si = circshift(s,-c_i_prev);  

%Target point defined as np_head points wrt to closest point -> L1
s_targ = si(np_ahead);   
[xT,yT,zT] = gen_path8(s_targ,e1,e2,pc,R);      %Generate the target point
target_p = [xT,yT,zT];

%Calculate the distance btw current aircraft pos and target point
d_l1 = sqrt((xT - a_posW(1))^2 + (yT - a_posW(2))^2 +(zT - a_posW(3))^2);

 end

== matlab function simL0_multiPath/Computer 1/State_flight controller ==
  data: switch_flag input; f_state output; trans_flag input; trac_flag input; state_prev input; state_prev output; state input; state output
% Flight computer controller

% switch_flag -> trigger from traction to retraction
% trans_flag  -> trigger from retraction to crossfligth
 

function [f_state,state_prev, state] = fcn(switch_flag,trans_flag, trac_flag, state_prev, state)

if state_prev == 1 && switch_flag == 1
    state = 2;
end

if state_prev == 2 && trans_flag == 1
   state = 1;
end

if state_prev == 3 && trac_flag == 1
   state = 1;
end

state_prev = state;
f_state = state;
end

== matlab function simL0_multiPath/Controls/ FlightControl/Switch_flystate/MATLAB Function ==
  data: s input; r output; t output; pathparam parameter
function [r , t ]= trig_switch_state(s, pathparam)
    if pathparam.isCircle
        if s >= 3*pi/2 && s < 5*pi/3  
            r = 1;
        else 
            r = 0;
        end 

        if s >= pi/2 && s < 3*pi/2
            t = 1;
        else 
            t = 0;
        end 
    else
        k = pathparam.direction;
        if k<0 % up loop
            if s >pi/2 && s< 2*pi/3  
                r = 1;
            else 
                r = 0;
            end 

            if s >= 4*pi/3 && s < 2*pi
                t = 1;
            else 
                t = 0;
            end
        else % down loop
            if s >0 && s< pi/10  %u >= 5*pi/3 && u < 2*pi 
                r = 1;
            else 
                r = 0;
            end 

            if s >= pi/2 && s < 3*pi/2
                t = 1;
            else 
                t = 0;
            end 
        end
    end
end

== matlab function simL0_multiPath/aerodynamic forces/HLW/Switch Solver Compiled ==
  data: input input double; out output double size=[8,1]; MegAWESkite parameter; ENVMT parameter
%% switch sim after runtime

function out = simpleAero(input, MegAWESkite, ENVMT)

    % MAIN LOOK-UP TABLE
    alpha = atan2(input(3),input(1));
    
    alpha_damp = atan2((MegAWESkite.elevator.momentArm+...
        MegAWESkite.elevator.chord*0.25+MegAWESkite.cog(1))*input(5),...
        input(1));

    q = 0.5*ENVMT.rhos*input(1)^2;
    
    beta = atan2(input(2),input(1));

    % ELEVATOR 
    % elevator: all moving horizontal stabilizer
    alpha_el = (MegAWESkite.elevator.alpha0 + alpha + alpha_damp + ...
        input(7)*pi/180)*180/pi;
    
    max_data_aoa = max(MegAWESkite.aero.elevator.alpha);
    min_data_aoa = min(MegAWESkite.aero.elevator.alpha);
    if alpha_el > max_data_aoa
        alpha_el = max_data_aoa;
    elseif alpha_el < min_data_aoa
        alpha_el = min_data_aoa;
    end
    alpha_aero = MegAWESkite.aero.elevator.alpha;
    cl = MegAWESkite.aero.elevator.cL;
    cd = MegAWESkite.aero.elevator.cD;
    cm = MegAWESkite.aero.elevator.cM;

    F_L_el = interp1(alpha_aero, cl, alpha_el,'spline')*q*MegAWESkite.elevator.areaSurface;
    F_D_el = interp1(alpha_aero, cd, alpha_el,'spline')*q*MegAWESkite.elevator.areaSurface;
    
    F_x_s = -F_D_el*cos(alpha)*cos(beta) + F_L_el*sin(alpha)*cos(beta);
%     F_y_s = -F_D_el*cos(alpha)*sin(beta) - F_L_el*sin(alpha)*sin(beta);
    F_y_s = 0;
    F_z_s = -F_L_el*cos(alpha);%+F_D_el*sin(alpha);

    M_x_s = 0;
%     M_el = interp1(alpha_aero, cm, alpha_el,'spline')*q*MegAWESkite.elevator.areaSurface*MegAWESkite.elevator.chord;
    M_el=0;
    M_y_s = M_el - F_L_el*(MegAWESkite.elevator.momentArm+...
        MegAWESkite.elevator.chord*0.25+MegAWESkite.cog(1));
    M_z_s = 0;

    out = [F_x_s, F_y_s, F_z_s, M_x_s, M_y_s, M_z_s, 0, 0]';

end

== matlab function simL0_multiPath/aerodynamic forces/SLW/Switch Solver Compiled ==
  data: input input double; out output double size=[8,1]; MegAWESkite parameter; ENVMT parameter
%% switch sim after runtime

function out = simpleAero(input, MegAWESkite, ENVMT)

    % MAIN LOOK-UP TABLE
    alpha = atan2(input(3),input(1));

    q = 0.5*ENVMT.rhos*input(1)^2;

    beta = atan2(input(2),input(1));

    beta_damp = -atan2((MegAWESkite.rudder.momentArm + ...
        MegAWESkite.rudder.chord*0.25+MegAWESkite.cog(1))*input(6),input(1));

    % vertical stabilizer
    alpha_vs = (MegAWESkite.rudder.alpha0 + beta_damp + beta)*180/pi+input(7);

    max_data_aoa = max(MegAWESkite.aero.rudder.alpha);
    min_data_aoa = min(MegAWESkite.aero.rudder.alpha);
    if alpha_vs > max_data_aoa
        alpha_vs = max_data_aoa;
    elseif alpha_vs < min_data_aoa
        alpha_vs = min_data_aoa;
    end
    
    alpha_aero = MegAWESkite.aero.rudder.alpha;
    cl = MegAWESkite.aero.rudder.cL;
    cd = MegAWESkite.aero.rudder.cD;
    cm = MegAWESkite.aero.rudder.cM;
    F_L_vs = 2*interp1(alpha_aero, cl, alpha_vs,'spline') * q * ...
        MegAWESkite.rudder.areaSurface;
    F_D_vs = 2*interp1(alpha_aero, cd, alpha_vs,'spline') * q * ...
        MegAWESkite.rudder.areaSurface;

    F_x_s = -F_D_vs*cos(alpha)*cos(beta);%-F_L_vs*cos(alpha)*sin(beta);
    F_y_s = -F_L_vs*cos(beta);%-F_D_vs*sin(beta);
    F_z_s = 0;% F_L_vs*sin(beta)*sin(alpha)+F_D_vs*cos(beta)*sin(alpha);

    M_x_s = 0;
    M_y_s = 0;
%     M_vs = 2*interp1(alpha_aero, cm, alpha_vs,'spline')*q*MegAWESkite.rudder.areaSurface*MegAWESkite.rudder.chord;
    M_vs = 0;
    M_z_s = M_vs+F_L_vs*(MegAWESkite.rudder.momentArm+...
        MegAWESkite.rudder.chord*0.25+...
        MegAWESkite.cog(1));

    out = [F_x_s, F_y_s, F_z_s, M_x_s, M_y_s, M_z_s,0,0]';

end

== matlab function simL0_multiPath/Controls/ FlightControl/traction/Heading_angle1 ==
  data: v_vel input; n output; v_targ input; v_tan output
% Function paht_tan_ang:

% It calculates the path angle on the tangential plane on the
% sphere knowing the projection on NE plane of the velocity (v_vel)
% and target (vector v)

function [n, v_tan]  = path_tan_ang(v_vel,v_targ)

%consider only the component on the NE plane
vec_vt = [v_vel(2) v_vel(3)];     %vector_velocity on tangential plane yz
vec_t = [v_targ(2) v_targ(3)];    %v_target


n = atan2(det([vec_vt; vec_t]), dot(vec_vt,vec_t));   
% the angle n is define btw velocity and target vector such as:
% + positive --> rotate vel clock-wise to reach target vect
% - negative --> rotate vel anti-clockwise to reach target vect

v_tan = sqrt(v_vel(2)*v_vel(2) +v_vel(3)*v_vel(3));

%Try another method to calculate the angle btw two vectors
% dot_product = dot(vec_vt, vec_t);
% 
% length_v = norm(vec_vt);
% length_t = norm(vec_t);
% 
% n1 = acos(dot_product / (length_v * length_t));

end
